simulink subsystem "Websockets_EchoClient"  (R2022b)
settings: Solver=VariableStepAuto  StartTime=0.0  StopTime=10.0  RelTol=1e-3
model mask{mi_ip=mi_ip, mi_port=mi_port}
  mask prompts: mi_ip "Server IP"; mi_port "Server Port"
libraries: slrealtimeiplib x2
settings Model: Creator=ramuj  LastModifiedBy=ramuj

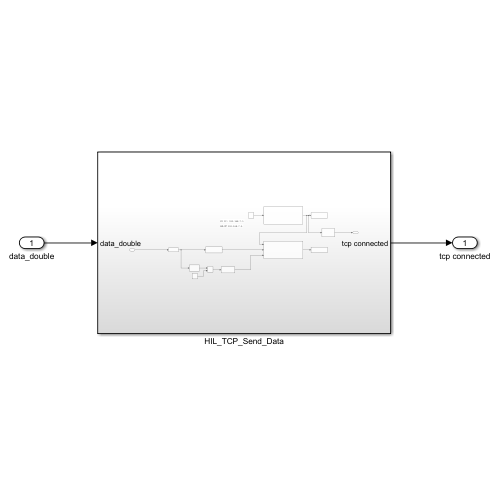
[thumbnail: Simulink's stored preview of the top-level diagram]
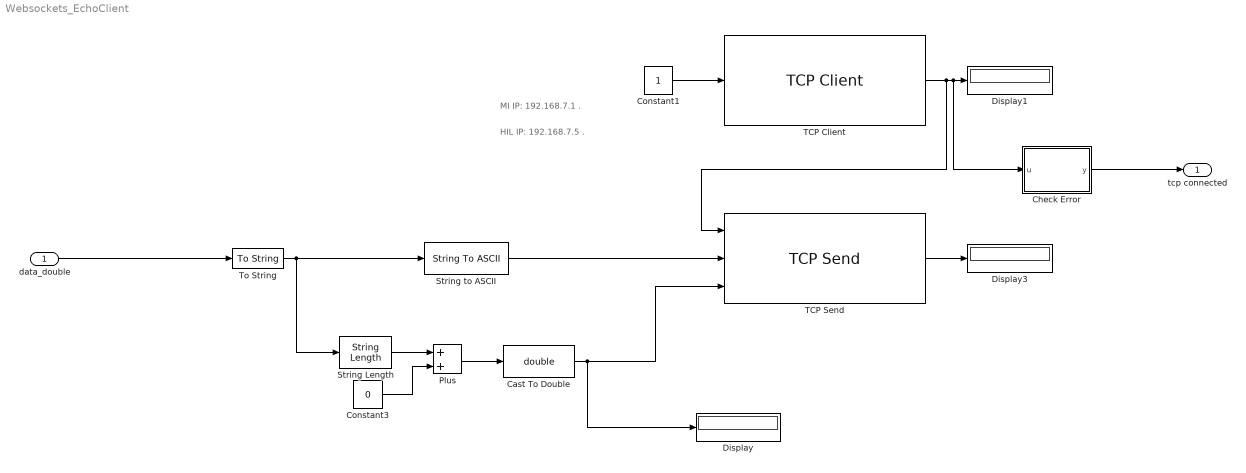
== system Websockets_EchoClient ==
  note: MI IP: 192.168.7.1 .
  note: HIL IP: 192.168.7.5 .
  data_double : Inport
  Cast To Double : DataTypeConversion  OutDataTypeStr=double  SaturateOnIntegerOverflow=off  RndMeth=Floor
  Check Error : MATLAB Function  TreatAsAtomicUnit=on
  Constant1 : Constant
  Constant3 : Constant  Value=0
  Display : Display
  Display1 : Display
  Display3 : Display
  Plus : Sum
  String Length : StringLength
  String to ASCII : StringToASCII
  TCP Client : slrealtimeiplib/TCP Client  Priority=-1  useHostTargetConn=off  remoteAddress=mi_ip  remotePort=mi_port
  TCP Send : slrealtimeiplib/TCP Send  socketAddPortVal=Client: 0.0.0.0:0  sampleTime=-1
  To String : ToString
  tcp connected : Outport
  wires:
  String Length/1 -> Plus/1
  Cast To Double/1 -> TCP Send/3, Display/1
  Plus/1 -> Cast To Double/1
  Check Error/1(y) -> tcp connected/1
  To String/1 -> String Length/1, String to ASCII/1
  Constant1/1 -> TCP Client/1
  TCP Client/1 -> TCP Send/1, Check Error/1(u), Display1/1
  data_double/1 -> To String/1
  TCP Send/1 -> Display3/1
  String to ASCII/1 -> TCP Send/2
  Constant3/1 -> Plus/2

== matlab function Websockets_EchoClient/Check Error ==
  data: u input; y output
function y = fcn(u)

    if(u == 1)
        y = "Connected";
    else 
        y = "Error";
    end
end
